simulink model "Manipulator_4DOF_dynamics_001"  (R2021b)
settings: Solver=VariableStepAuto  StartTime=0.0  StopTime=10.0  RelTol=1e-3
settings Model: Creator=rusla  LastModifiedBy=rusla

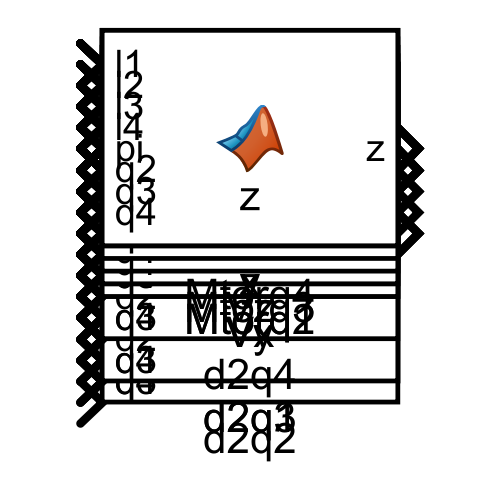
[thumbnail: Simulink's stored preview of the top-level diagram]
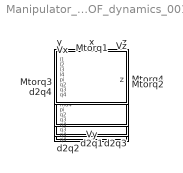
== system Manipulator_4DOF_dynamics_001 ==
  Mtorq1 : MATLAB Function  TreatAsAtomicUnit=on
  Mtorq2 : MATLAB Function  TreatAsAtomicUnit=on
  Mtorq3 : MATLAB Function  TreatAsAtomicUnit=on
  Mtorq4 : MATLAB Function  TreatAsAtomicUnit=on
  Vx : MATLAB Function  TreatAsAtomicUnit=on
  Vy : MATLAB Function  TreatAsAtomicUnit=on
  Vz : MATLAB Function  TreatAsAtomicUnit=on
  d2q1 : MATLAB Function  TreatAsAtomicUnit=on
  d2q2 : MATLAB Function  TreatAsAtomicUnit=on
  d2q3 : MATLAB Function  TreatAsAtomicUnit=on
  d2q4 : MATLAB Function  TreatAsAtomicUnit=on
  x : MATLAB Function  TreatAsAtomicUnit=on
  y : MATLAB Function  TreatAsAtomicUnit=on
  z : MATLAB Function  TreatAsAtomicUnit=on

== matlab function Manipulator_4DOF_dynamics_001/Vx ==
  data: dq1 input; Vx output; dq2 input; dq3 input; dq4 input; l2 input; l3 input; l4 input; pi input; q1 input; q2 input; q3 input; q4 input
function Vx = Vx(dq1,dq2,dq3,dq4,l2,l3,l4,pi,q1,q2,q3,q4)
%#codegen

%    This function was generated by the Symbolic Math Toolbox version 9.0.
%    11-May-2022 22:38:02

t2 = cos(q1);
t3 = cos(q2);
t4 = cos(q3);
t5 = cos(q4);
t6 = sin(q1);
t7 = sin(q2);
t8 = sin(q3);
t9 = sin(q4);
t14 = pi./2.0;
t10 = t2.*t3;
t11 = t2.*t7;
t12 = t3.*t6;
t13 = t6.*t7;
t15 = cos(t14);
t16 = t10.*t15;
t17 = t11.*t15;
t18 = t12.*t15;
t19 = t13.*t15;
t20 = -t17;
t21 = -t18;
t22 = t10+t19;
t23 = t13+t16;
t24 = t11+t21;
t25 = t12+t20;
t26 = t8.*t22;
t27 = t8.*t23;
t28 = t4.*t22;
t29 = t8.*t24;
t30 = t4.*t24;
t31 = t4.*t25;
t32 = -t30;
t33 = t27+t31;
t34 = t28+t29;
t35 = t26+t32;
t36 = t9.*t34;
t37 = l3.*t35;
t38 = t5.*t35;
t39 = t36+t38;
t40 = l4.*t39;
Vx = -dq3.*(t37+t40)-dq4.*t40+dq2.*(t37+t40-l2.*t24)-dq1.*(l4.*(t5.*t33+t9.*(t4.*t23-t8.*t25))+l2.*t25+l3.*t33);

== matlab function Manipulator_4DOF_dynamics_001/Vy ==
  data: dq1 input; Vy output; dq2 input; dq3 input; dq4 input; l2 input; l3 input; l4 input; pi input; q1 input; q2 input; q3 input; q4 input
function Vy = Vy(dq1,dq2,dq3,dq4,l2,l3,l4,pi,q1,q2,q3,q4)
%#codegen

%    This function was generated by the Symbolic Math Toolbox version 9.0.
%    11-May-2022 22:38:03

t2 = cos(q1);
t3 = cos(q2);
t4 = cos(q3);
t5 = cos(q4);
t6 = sin(q1);
t7 = sin(q2);
t8 = sin(q3);
t9 = sin(q4);
t14 = pi./2.0;
t10 = t2.*t3;
t11 = t2.*t7;
t12 = t3.*t6;
t13 = t6.*t7;
t15 = cos(t14);
t16 = t10.*t15;
t17 = t11.*t15;
t18 = t12.*t15;
t19 = t13.*t15;
t20 = -t17;
t21 = -t18;
t22 = t10+t19;
t23 = t13+t16;
t24 = t11+t21;
t25 = t12+t20;
t26 = t8.*t23;
t27 = t4.*t22;
t28 = t4.*t23;
t29 = t8.*t24;
t30 = t8.*t25;
t31 = t4.*t25;
t32 = -t28;
t33 = t26+t31;
t34 = t27+t29;
t35 = t30+t32;
t37 = -l3.*(t28-t30);
t38 = -t5.*(t28-t30);
t36 = t9.*t33;
t39 = t36+t38;
t40 = l4.*t39;
Vy = -dq3.*(t37+t40)-dq4.*t40-dq2.*(-t40+l2.*t23+l3.*(t28-t30))+dq1.*(l4.*(t5.*t34+t9.*(t4.*t24-t8.*t22))+l2.*t22+l3.*t34);

== matlab function Manipulator_4DOF_dynamics_001/Vz ==
  data: dq2 input; Vz output; dq3 input; dq4 input; l2 input; l3 input; l4 input; pi input; q2 input; q3 input; q4 input
function Vz = Vz(dq2,dq3,dq4,l2,l3,l4,pi,q2,q3,q4)
%#codegen

%    This function was generated by the Symbolic Math Toolbox version 9.0.
%    11-May-2022 22:38:04

t2 = -q2;
t3 = -q3;
t4 = q2+t3;
t6 = q3+q4+t2;
t5 = cos(t4);
t7 = cos(t6);
Vz = sin(pi./2.0).*(dq2.*l2.*cos(q2)+dq2.*l3.*t5-dq3.*l3.*t5+dq2.*l4.*t7-dq3.*l4.*t7-dq4.*l4.*t7);

== matlab function Manipulator_4DOF_dynamics_001/Mtorq1 ==
  data: Fx input; Mtorq1 output; Fy input; Mfi input; l2 input; l3 input; l4 input; pi input; q1 input; q2 input; q3 input; q4 input
function Mtorq1 = Mtorq1(Fx,Fy,Mfi,l2,l3,l4,pi,q1,q2,q3,q4)
%#codegen

%    This function was generated by the Symbolic Math Toolbox version 9.0.
%    11-May-2022 22:38:05

t2 = cos(q1);
t3 = cos(q2);
t4 = cos(q3);
t5 = cos(q4);
t6 = sin(q1);
t7 = sin(q2);
t8 = sin(q3);
t9 = sin(q4);
t14 = pi./2.0;
t10 = t2.*t3;
t11 = t2.*t7;
t12 = t3.*t6;
t13 = t6.*t7;
t15 = cos(t14);
t16 = t10.*t15;
t17 = t11.*t15;
t18 = t12.*t15;
t19 = t13.*t15;
t20 = -t17;
t21 = -t18;
t22 = t10+t19;
t23 = t13+t16;
t24 = t11+t21;
t25 = t12+t20;
t26 = t8.*t23;
t27 = t4.*t22;
t28 = t8.*t24;
t29 = t4.*t25;
t30 = t26+t29;
t31 = t27+t28;
Mtorq1 = Mfi-Fx.*(l4.*(t5.*t30+t9.*(t4.*t23-t8.*t25))+l2.*t25+l3.*t30)+Fy.*(l4.*(t5.*t31+t9.*(t4.*t24-t8.*t22))+l2.*t22+l3.*t31);

== matlab function Manipulator_4DOF_dynamics_001/Mtorq2 ==
  data: Fx input; Mtorq2 output; Fy input; Fz input; l2 input; l3 input; l4 input; pi input; q1 input; q2 input; q3 input; q4 input
function Mtorq2 = Mtorq2(Fx,Fy,Fz,l2,l3,l4,pi,q1,q2,q3,q4)
%#codegen

%    This function was generated by the Symbolic Math Toolbox version 9.0.
%    11-May-2022 22:38:06

t2 = cos(q1);
t3 = cos(q2);
t4 = cos(q3);
t5 = cos(q4);
t6 = sin(q1);
t7 = sin(q2);
t8 = sin(q3);
t9 = sin(q4);
t10 = -q3;
t15 = pi./2.0;
t11 = t2.*t3;
t12 = t2.*t7;
t13 = t3.*t6;
t14 = t6.*t7;
t16 = cos(t15);
t17 = sin(t15);
t18 = q2+t10;
t19 = t11.*t16;
t20 = t12.*t16;
t21 = t13.*t16;
t22 = t14.*t16;
t23 = -t20;
t24 = -t21;
t25 = t11+t22;
t26 = t14+t19;
t27 = t12+t24;
t28 = t13+t23;
t29 = t8.*t25;
t30 = t4.*t26;
t31 = t8.*t28;
t32 = t4.*t27;
t33 = -t30;
t34 = -t32;
t36 = t31+t33;
t35 = t29+t34;
Mtorq2 = -Fy.*(l2.*t26+l4.*(t5.*(t30-t31)-t9.*(t4.*t28+t8.*t26))+l3.*(t30-t31))+Fx.*(l4.*(t5.*t35+t9.*(t4.*t25+t8.*t27))-l2.*t27+l3.*t35)+Fz.*(l4.*(t5.*t17.*cos(t18)+t9.*t17.*sin(t18))+l3.*(t3.*t4.*t17+t7.*t8.*t17)+l2.*t3.*t17);

== matlab function Manipulator_4DOF_dynamics_001/Mtorq3 ==
  data: Fx input; Mtorq3 output; Fy input; Fz input; l3 input; l4 input; pi input; q1 input; q2 input; q3 input; q4 input
function Mtorq3 = Mtorq3(Fx,Fy,Fz,l3,l4,pi,q1,q2,q3,q4)
%#codegen

%    This function was generated by the Symbolic Math Toolbox version 9.0.
%    11-May-2022 22:38:07

t2 = cos(q1);
t3 = cos(q2);
t4 = cos(q3);
t5 = cos(q4);
t6 = sin(q1);
t7 = sin(q2);
t8 = sin(q3);
t9 = sin(q4);
t10 = -q3;
t15 = pi./2.0;
t11 = t2.*t3;
t12 = t2.*t7;
t13 = t3.*t6;
t14 = t6.*t7;
t16 = cos(t15);
t17 = sin(t15);
t18 = q2+t10;
t19 = t11.*t16;
t20 = t12.*t16;
t21 = t13.*t16;
t22 = t14.*t16;
t23 = -t20;
t24 = -t21;
t25 = t11+t22;
t26 = t14+t19;
t27 = t12+t24;
t28 = t13+t23;
t29 = t8.*t25;
t30 = t4.*t26;
t31 = t8.*t28;
t32 = t4.*t27;
t33 = -t30;
t34 = -t32;
t36 = t31+t33;
t35 = t29+t34;
Mtorq3 = -Fz.*(l4.*(t5.*t17.*cos(t18)+t9.*t17.*sin(t18))+l3.*(t3.*t4.*t17+t7.*t8.*t17))-Fx.*(l4.*(t5.*t35+t9.*(t4.*t25+t8.*t27))+l3.*t35)+Fy.*(l4.*(t5.*(t30-t31)-t9.*(t4.*t28+t8.*t26))+l3.*(t30-t31));

== matlab function Manipulator_4DOF_dynamics_001/Mtorq4 ==
  data: Fx input; Mtorq4 output; Fy input; Fz input; l4 input; pi input; q1 input; q2 input; q3 input; q4 input
function Mtorq4 = Mtorq4(Fx,Fy,Fz,l4,pi,q1,q2,q3,q4)
%#codegen

%    This function was generated by the Symbolic Math Toolbox version 9.0.
%    11-May-2022 22:38:08

t2 = cos(q1);
t3 = cos(q2);
t4 = cos(q3);
t5 = cos(q4);
t6 = sin(q1);
t7 = sin(q2);
t8 = sin(q3);
t9 = sin(q4);
t10 = -q3;
t15 = pi./2.0;
t11 = t2.*t3;
t12 = t2.*t7;
t13 = t3.*t6;
t14 = t6.*t7;
t16 = cos(t15);
t17 = sin(t15);
t18 = q2+t10;
t19 = t11.*t16;
t20 = t12.*t16;
t21 = t13.*t16;
t22 = t14.*t16;
t23 = -t20;
t24 = -t21;
t25 = t11+t22;
t26 = t14+t19;
t27 = t12+t24;
t28 = t13+t23;
Mtorq4 = -Fz.*l4.*(t5.*t17.*cos(t18)+t9.*t17.*sin(t18))+Fx.*l4.*(t5.*(t4.*t27-t8.*t25)-t9.*(t4.*t25+t8.*t27))+Fy.*l4.*(t5.*(t4.*t26-t8.*t28)-t9.*(t4.*t28+t8.*t26));

== matlab function Manipulator_4DOF_dynamics_001/x ==
  data: l2 input; x output; l3 input; l4 input; pi input; q1 input; q2 input; q3 input; q4 input
function x = x(l2,l3,l4,pi,q1,q2,q3,q4)
%#codegen

%    This function was generated by the Symbolic Math Toolbox version 9.0.
%    11-May-2022 22:38:09

t2 = cos(q1);
t3 = cos(q2);
t4 = cos(q3);
t5 = sin(q1);
t6 = sin(q2);
t7 = sin(q3);
t10 = pi./2.0;
t8 = t2.*t3;
t9 = t2.*t6;
t11 = cos(t10);
t12 = t3.*t5.*t11;
t13 = t5.*t6.*t11;
t14 = -t12;
t15 = t8+t13;
t16 = t9+t14;
t17 = t4.*t15;
t18 = t7.*t16;
t19 = t17+t18;
x = l4.*(sin(q4).*(t4.*t16-t7.*t15)+t19.*cos(q4))+l2.*t15+l3.*t19;

== matlab function Manipulator_4DOF_dynamics_001/d2q2 ==
  data: B input; d2q2 output; dq1 input; dq2 input; dq3 input; dq4 input; g input; l2 input; l3 input; l4 input; m2 input; m3 input; m4 input; mu2 input; pi input; q2 input; q3 input; q4 input
function d2q2 = d2q2(B,dq1,dq2,dq3,dq4,g,l2,l3,l4,m2,m3,m4,mu2,pi,q2,q3,q4)
%#codegen

%    This function was generated by the Symbolic Math Toolbox version 9.0.
%    11-May-2022 22:37:59

t2 = cos(q2);
t3 = sin(q3);
t4 = sin(q4);
t5 = B+q4;
t6 = q3+q4;
t7 = B.*2.0;
t8 = dq1.^2;
t9 = dq3.^2;
t10 = dq4.^2;
t11 = l2.^2;
t12 = l3.^2;
t13 = l4.^2;
t14 = q2.*2.0;
t15 = q3.*2.0;
t16 = q4.*2.0;
t21 = -pi;
t22 = -q2;
t24 = -q3;
t26 = -q4;
t28 = pi./2.0;
t17 = sin(t14);
t18 = q3+t5;
t19 = sin(t5);
t20 = sin(t6);
t23 = -t14;
t25 = -t15;
t27 = pi+t14;
t31 = cos(t28);
t32 = sin(t28);
t34 = q2+t24;
t38 = t14+t24;
t29 = sin(t18);
t30 = sin(t27);
t33 = pi+t23;
t35 = cos(t34);
t39 = t14+t25;
t41 = t24+t27;
t43 = t25+t27;
t44 = sin(t38);
t36 = q3+t33;
t37 = sin(t33);
t42 = t15+t33;
t45 = sin(t39);
t46 = sin(t41);
t48 = sin(t43);
t40 = sin(t36);
t47 = sin(t42);
et1 = mu2.*4.0-(m2.*t8.*t11.*t17)./3.0-m3.*t8.*t11.*t17-m4.*t8.*t11.*t17+(m2.*t8.*t11.*t30)./6.0+(m3.*t8.*t11.*t30)./2.0+(m4.*t8.*t11.*t30)./2.0-(m2.*t8.*t11.*t37)./6.0-(m3.*t8.*t11.*t37)./2.0-(m4.*t8.*t11.*t37)./2.0-(m3.*t8.*t12.*t45)./3.0-m4.*t8.*t12.*t45-(m3.*t8.*t12.*t47)./6.0+(m3.*t8.*t12.*t48)./6.0-(m4.*t8.*t12.*t47)./2.0+(m4.*t8.*t12.*t48)./2.0+(m4.*t8.*t13.*sin(t5.*2.0+t15+t23))./3.0+(m4.*t8.*t13.*sin(t6+t18+t21+t23))./2.0-(m4.*t8.*t13.*sin(t5.*2.0+t15+t21+t23))./6.0+m4.*t8.*t13.*sin(t6.*2.0+t23)+(m4.*t8.*t13.*sin(t6.*-2.0+t27))./2.0;
et2 = m4.*t8.*t13.*sin(t6.*2.0+t33).*(-1.0./2.0)-(m4.*t8.*t13.*sin(t5.*2.0+t42))./6.0-m4.*t8.*t13.*sin(t6+t18+t23)+(m4.*t8.*t13.*sin(t6+t18+t33))./2.0+l2.*l4.*m4.*t8.*sin(-t6+t27)+l3.*l4.*m4.*t8.*sin(-t6+t41)+l3.*l4.*m4.*t8.*sin(q3+t6+t23).*2.0-l3.*l4.*m4.*t8.*sin(t5+t15+t23)+(l2.*l4.*m4.*t8.*sin(t18+t21+t23))./2.0-g.*l2.*m2.*t2.*t32.*2.0-g.*l2.*m3.*t2.*t32.*4.0-g.*l2.*m4.*t2.*t32.*4.0-g.*l3.*m3.*t32.*t35.*2.0-g.*l3.*m4.*t32.*t35.*4.0-l2.*l3.*m3.*t3.*t9.*2.0-l2.*l3.*m4.*t3.*t9.*4.0-l3.*l4.*m4.*t4.*t10.*4.0-l2.*l4.*m4.*t9.*t20.*4.0-l2.*l4.*m4.*t10.*t20.*4.0+l3.*l4.*m4.*t10.*t19.*2.0;
et3 = l2.*l4.*m4.*t9.*t29.*2.0+l2.*l4.*m4.*t10.*t29.*2.0-(l2.*l3.*m3.*t8.*t40)./2.0-l2.*l3.*m4.*t8.*t40-l2.*l3.*m3.*t8.*t44-l2.*l3.*m4.*t8.*t44.*2.0+(l2.*l3.*m3.*t8.*t46)./2.0+l2.*l3.*m4.*t8.*t46+(l3.*l4.*m4.*t8.*sin(t5+t15+t21+t23))./2.0-g.*l4.*m4.*t32.*cos(t6+t22).*4.0+g.*l4.*m4.*t32.*cos(t18+t22).*2.0+l2.*l4.*m4.*t8.*sin(t6+t23).*2.0-l2.*l4.*m4.*t8.*sin(t6+t33)-l2.*l4.*m4.*t8.*sin(t18+t23)-l3.*l4.*m4.*t8.*sin(t6+t36)+(l3.*l4.*m4.*t8.*sin(t5+t42))./2.0+(l2.*l4.*m4.*t8.*sin(t18+t33))./2.0+dq2.*dq3.*l2.*l3.*m3.*t3.*4.0+dq2.*dq3.*l2.*l3.*m4.*t3.*8.0+dq2.*dq4.*l3.*l4.*m4.*t4.*8.0;
et4 = dq3.*dq4.*l3.*l4.*m4.*t4.*-8.0+dq2.*dq3.*l2.*l4.*m4.*t20.*8.0+dq2.*dq4.*l2.*l4.*m4.*t20.*8.0-dq2.*dq4.*l3.*l4.*m4.*t19.*4.0-dq3.*dq4.*l2.*l4.*m4.*t20.*8.0+dq3.*dq4.*l3.*l4.*m4.*t19.*4.0-dq2.*dq3.*l2.*l4.*m4.*t29.*4.0-dq2.*dq4.*l2.*l4.*m4.*t29.*4.0+dq3.*dq4.*l2.*l4.*m4.*t29.*4.0-dq1.*dq3.*l2.*l3.*m3.*t3.*t31.*4.0-dq1.*dq3.*l2.*l3.*m4.*t3.*t31.*8.0-dq1.*dq4.*l3.*l4.*m4.*t4.*t31.*8.0-dq1.*dq3.*l2.*l4.*m4.*t20.*t31.*8.0-dq1.*dq4.*l2.*l4.*m4.*t20.*t31.*8.0+dq1.*dq4.*l3.*l4.*m4.*t19.*t31.*4.0+dq1.*dq3.*l2.*l4.*m4.*t29.*t31.*4.0+dq1.*dq4.*l2.*l4.*m4.*t29.*t31.*4.0;
d2q2 = et1+et2+et3+et4;

== matlab function Manipulator_4DOF_dynamics_001/y ==
  data: l2 input; y output; l3 input; l4 input; pi input; q1 input; q2 input; q3 input; q4 input
function y = y(l2,l3,l4,pi,q1,q2,q3,q4)
%#codegen

%    This function was generated by the Symbolic Math Toolbox version 9.0.
%    11-May-2022 22:38:10

t2 = cos(q1);
t3 = cos(q2);
t4 = cos(q3);
t5 = sin(q1);
t6 = sin(q2);
t7 = sin(q3);
t10 = pi./2.0;
t8 = t3.*t5;
t9 = t5.*t6;
t11 = cos(t10);
t12 = t2.*t3.*t11;
t13 = t2.*t6.*t11;
t14 = -t13;
t15 = t9+t12;
t16 = t8+t14;
t17 = t7.*t15;
t18 = t4.*t16;
t19 = t17+t18;
y = l4.*(sin(q4).*(t4.*t15-t7.*t16)+t19.*cos(q4))+l2.*t16+l3.*t19;

== matlab function Manipulator_4DOF_dynamics_001/z ==
  data: l1 input; z output; l2 input; l3 input; l4 input; pi input; q2 input; q3 input; q4 input
function z = z(l1,l2,l3,l4,pi,q2,q3,q4)
%#codegen

%    This function was generated by the Symbolic Math Toolbox version 9.0.
%    11-May-2022 22:38:10

t2 = sin(q2);
t3 = -q3;
t4 = pi./2.0;
t5 = sin(t4);
t6 = q2+t3;
z = l1+l4.*(t5.*cos(q4).*sin(t6)-t5.*cos(t6).*sin(q4))+l3.*(t2.*t5.*cos(q3)-t5.*cos(q2).*sin(q3))+l2.*t2.*t5;

== matlab function Manipulator_4DOF_dynamics_001/d2q1 ==
  data: B input; d2q1 output; dq1 input; dq2 input; dq3 input; dq4 input; l2 input; l3 input; l4 input; m2 input; m3 input; m4 input; mu1 input; pi input; q2 input; q3 input; q4 input
function d2q1 = d2q1(B,dq1,dq2,dq3,dq4,l2,l3,l4,m2,m3,m4,mu1,pi,q2,q3,q4)
%#codegen

%    This function was generated by the Symbolic Math Toolbox version 9.0.
%    11-May-2022 22:37:55

t2 = sin(q3);
t3 = sin(q4);
t4 = B+q4;
t5 = pi+q3;
t6 = q3+q4;
t7 = B.*2.0;
t8 = dq3.^2;
t9 = l2.^2;
t10 = l3.^2;
t11 = l4.^2;
t12 = q2.*2.0;
t13 = q3.*2.0;
t14 = q4.*2.0;
t21 = -pi;
t23 = -q3;
t25 = -q4;
t29 = pi./2.0;
t15 = sin(t12);
t16 = q3+t4;
t17 = sin(t4);
t18 = q4+t5;
t19 = sin(t5);
t20 = sin(t6);
t22 = -t12;
t24 = -t13;
t26 = -t14;
t28 = pi+t12;
t30 = t4+t5;
t35 = pi+t23;
t36 = -t29;
t38 = t6+t21;
t42 = q3+t29;
t43 = q4+t29;
t44 = t12+t23;
t46 = t6+t29;
t55 = t4+t29;
t82 = t23+t29;
t83 = t25+t29;
t27 = sin(t18);
t31 = sin(t16);
t32 = sin(t28);
t33 = sin(t30);
t34 = pi+t22;
t37 = t5+t22;
t39 = t6+t22;
t41 = sin(t35);
t45 = t12+t24;
t47 = sin(t42);
t48 = sin(t43);
t49 = t16+t21;
t50 = t16+t22;
t51 = t18+t22;
t53 = sin(t38);
t56 = t6+t36;
t57 = t16+t29;
t58 = sin(t55);
t59 = t23+t28;
t61 = t24+t28;
t63 = sin(t44);
t65 = sin(t46);
t66 = t22+t30;
t69 = t4+t36;
t72 = t16+t36;
t75 = t4+t13+t22;
t87 = sin(t82);
t88 = sin(t83);
t96 = -t6+t28;
t40 = sin(t34);
t52 = sin(t37);
t54 = sin(t39);
t60 = q3+t37;
t62 = q3+t39;
t64 = sin(t45);
t67 = sin(t49);
t68 = sin(t50);
t70 = sin(t51);
t71 = sin(t66);
t73 = sin(t69);
t74 = sin(t56);
t76 = sin(t57);
t77 = t6+t37;
t78 = sin(t59);
t80 = sin(t61);
t84 = t16+t37;
t85 = sin(t75);
t89 = sin(t72);
t90 = t6+t39;
t91 = t16+t39;
t92 = t22+t49;
t93 = t18+t39;
t97 = -t6+t59;
t98 = -t6+t96;
t99 = t30+t39;
t103 = t4+t75;
t104 = t21+t75;
t105 = sin(t96);
t109 = t30+t50;
t113 = t38+t50;
t79 = sin(t60);
t81 = sin(t62);
t86 = sin(t77);
t94 = sin(t90);
t95 = sin(t84);
t100 = sin(t91);
t101 = sin(t92);
t102 = sin(t93);
t106 = sin(t97);
t107 = sin(t98);
t108 = sin(t99);
t110 = sin(t103);
t111 = sin(t104);
t112 = sin(t109);
t114 = sin(t113);
t115 = t21+t103;
t116 = sin(t115);
et1 = mu1.*4.0+dq4.^2.*l4.*m4.*cos(t29).*(l3.*t3.*2.0-l3.*t17+l2.*t20.*2.0-l2.*t31).*2.0+dq1.*dq2.*m2.*t9.*t15.*(2.0./3.0)+dq1.*dq2.*m3.*t9.*t15.*2.0+dq1.*dq2.*m4.*t9.*t15.*2.0-(dq1.*dq2.*m2.*t9.*t32)./3.0-dq1.*dq2.*m3.*t9.*t32-dq1.*dq2.*m4.*t9.*t32+(dq1.*dq2.*m2.*t9.*t40)./3.0+dq1.*dq2.*m3.*t9.*t40+dq1.*dq2.*m4.*t9.*t40+dq1.*dq2.*m3.*t10.*t64.*(2.0./3.0)+dq1.*dq2.*m4.*t10.*t64.*2.0-dq1.*dq3.*m3.*t10.*t64.*(2.0./3.0)-dq1.*dq3.*m4.*t10.*t64.*2.0+(dq1.*dq2.*m3.*t10.*t79)./3.0-(dq1.*dq2.*m3.*t10.*t80)./3.0+dq1.*dq2.*m4.*t10.*t79-(dq1.*dq3.*m3.*t10.*t79)./3.0-dq1.*dq2.*m4.*t10.*t80+(dq1.*dq3.*m3.*t10.*t80)./3.0-dq1.*dq3.*m4.*t10.*t79;
et2 = dq1.*dq3.*m4.*t10.*t80-dq1.*dq2.*m4.*t11.*t94.*2.0+dq1.*dq3.*m4.*t11.*t94.*2.0+dq1.*dq4.*m4.*t11.*t94.*2.0+dq1.*dq2.*m4.*t11.*t100.*2.0-dq1.*dq3.*m4.*t11.*t100.*2.0+dq1.*dq2.*m4.*t11.*t102-dq1.*dq4.*m4.*t11.*t100.*2.0-dq1.*dq3.*m4.*t11.*t102-dq1.*dq4.*m4.*t11.*t102-dq1.*dq2.*m4.*t11.*t107-dq1.*dq2.*m4.*t11.*t108+dq1.*dq3.*m4.*t11.*t107+dq1.*dq3.*m4.*t11.*t108+dq1.*dq4.*m4.*t11.*t107-dq1.*dq2.*m4.*t11.*t110.*(2.0./3.0)+dq1.*dq4.*m4.*t11.*t108+dq1.*dq3.*m4.*t11.*t110.*(2.0./3.0)+(dq1.*dq2.*m4.*t11.*t112)./3.0+dq1.*dq4.*m4.*t11.*t110.*(2.0./3.0)-(dq1.*dq3.*m4.*t11.*t112)./3.0-dq1.*dq2.*m4.*t11.*t114-(dq1.*dq4.*m4.*t11.*t112)./3.0+dq1.*dq3.*m4.*t11.*t114+(dq1.*dq2.*m4.*t11.*t116)./3.0+dq1.*dq4.*m4.*t11.*t114;
et3 = dq1.*dq3.*m4.*t11.*t116.*(-1.0./3.0)-(dq1.*dq4.*m4.*t11.*t116)./3.0+l2.*l3.*m3.*t8.*t47+l2.*l3.*m4.*t8.*t47.*2.0+l2.*l4.*m4.*t8.*t65.*2.0+l2.*l4.*m4.*t8.*t74.*2.0-l2.*l4.*m4.*t8.*t76-l2.*l3.*m3.*t8.*t87-l2.*l3.*m4.*t8.*t87.*2.0-l2.*l4.*m4.*t8.*t89+dq1.*dq4.*l3.*l4.*m4.*sin(pi+q4)-(dq1.*dq4.*l3.*l4.*m4.*sin(pi+t4))./2.0-dq1.*dq4.*l3.*l4.*m4.*sin(pi+t25)-(dq1.*dq4.*l3.*l4.*m4.*sin(t4+t21))./2.0+dq1.*dq3.*l2.*l3.*m3.*t2.*3.0+dq1.*dq3.*l2.*l3.*m4.*t2.*6.0+dq1.*dq4.*l3.*l4.*m4.*t3.*6.0+(dq1.*dq3.*l2.*l3.*m3.*t19)./2.0+dq1.*dq3.*l2.*l3.*m4.*t19-dq1.*dq4.*l3.*l4.*m4.*t17.*3.0+dq1.*dq3.*l2.*l4.*m4.*t20.*6.0+dq1.*dq4.*l2.*l4.*m4.*t20.*6.0;
et4 = dq1.*dq3.*l2.*l4.*m4.*t27+dq1.*dq4.*l2.*l4.*m4.*t27-dq1.*dq3.*l2.*l4.*m4.*t31.*3.0-dq1.*dq4.*l2.*l4.*m4.*t31.*3.0-(dq1.*dq3.*l2.*l4.*m4.*t33)./2.0-(dq1.*dq4.*l2.*l4.*m4.*t33)./2.0-(dq1.*dq3.*l2.*l3.*m3.*t41)./2.0-dq1.*dq3.*l2.*l3.*m4.*t41-dq2.*dq3.*l2.*l3.*m3.*t47.*2.0-dq2.*dq3.*l2.*l3.*m4.*t47.*4.0+dq1.*dq2.*l2.*l3.*m3.*t52+dq1.*dq2.*l2.*l3.*m4.*t52.*2.0-(dq1.*dq3.*l2.*l3.*m3.*t52)./2.0-dq1.*dq3.*l2.*l3.*m4.*t52-dq2.*dq4.*l3.*l4.*m4.*t48.*4.0+dq3.*dq4.*l3.*l4.*m4.*t48.*4.0-dq1.*dq2.*l2.*l4.*m4.*t54.*4.0+dq1.*dq3.*l2.*l4.*m4.*t53+dq1.*dq3.*l2.*l4.*m4.*t54.*2.0+dq1.*dq4.*l2.*l4.*m4.*t53+dq1.*dq4.*l2.*l4.*m4.*t54.*2.0+dq1.*dq2.*l2.*l3.*m3.*t63.*2.0+dq1.*dq2.*l2.*l3.*m4.*t63.*4.0;
et5 = -dq1.*dq3.*l2.*l3.*m3.*t63+dq2.*dq4.*l3.*l4.*m4.*t58.*2.0-dq1.*dq3.*l2.*l3.*m4.*t63.*2.0-dq3.*dq4.*l3.*l4.*m4.*t58.*2.0-dq2.*dq3.*l2.*l4.*m4.*t65.*4.0+dq1.*dq2.*l2.*l4.*m4.*t68.*2.0-(dq1.*dq3.*l2.*l4.*m4.*t67)./2.0-dq2.*dq4.*l2.*l4.*m4.*t65.*4.0-dq1.*dq3.*l2.*l4.*m4.*t68-(dq1.*dq4.*l2.*l4.*m4.*t67)./2.0+dq3.*dq4.*l2.*l4.*m4.*t65.*4.0+dq1.*dq2.*l2.*l4.*m4.*t70.*2.0-dq1.*dq4.*l2.*l4.*m4.*t68-dq1.*dq2.*l2.*l4.*m4.*t71-dq1.*dq3.*l2.*l4.*m4.*t70+(dq1.*dq3.*l2.*l4.*m4.*t71)./2.0-dq1.*dq4.*l2.*l4.*m4.*t70+(dq1.*dq4.*l2.*l4.*m4.*t71)./2.0-dq1.*dq2.*l2.*l3.*m3.*t78-dq2.*dq3.*l2.*l4.*m4.*t74.*4.0-dq1.*dq2.*l2.*l3.*m4.*t78.*2.0;
et6 = (dq1.*dq3.*l2.*l3.*m3.*t78)./2.0-dq2.*dq4.*l2.*l4.*m4.*t74.*4.0+dq2.*dq4.*l3.*l4.*m4.*t73.*2.0+dq1.*dq3.*l2.*l3.*m4.*t78+dq2.*dq3.*l2.*l4.*m4.*t76.*2.0+dq3.*dq4.*l2.*l4.*m4.*t74.*4.0-dq3.*dq4.*l3.*l4.*m4.*t73.*2.0+dq2.*dq4.*l2.*l4.*m4.*t76.*2.0-dq3.*dq4.*l2.*l4.*m4.*t76.*2.0-dq1.*dq2.*l3.*l4.*m4.*t81.*4.0+dq1.*dq3.*l3.*l4.*m4.*t81.*4.0+dq1.*dq4.*l3.*l4.*m4.*t81.*2.0+dq1.*dq2.*l3.*l4.*m4.*t85.*2.0+dq1.*dq2.*l3.*l4.*m4.*t86.*2.0-dq1.*dq3.*l3.*l4.*m4.*t85.*2.0+dq2.*dq3.*l2.*l3.*m3.*t87.*2.0-dq1.*dq3.*l3.*l4.*m4.*t86.*2.0-dq1.*dq4.*l3.*l4.*m4.*t85+dq2.*dq3.*l2.*l3.*m4.*t87.*4.0-dq1.*dq4.*l3.*l4.*m4.*t86+dq2.*dq3.*l2.*l4.*m4.*t89.*2.0+dq2.*dq4.*l2.*l4.*m4.*t89.*2.0+dq2.*dq4.*l3.*l4.*m4.*t88.*4.0;
et7 = dq3.*dq4.*l2.*l4.*m4.*t89.*-2.0-dq3.*dq4.*l3.*l4.*m4.*t88.*4.0-dq1.*dq2.*l3.*l4.*m4.*t95+dq1.*dq3.*l3.*l4.*m4.*t95+(dq1.*dq4.*l3.*l4.*m4.*t95)./2.0-dq1.*dq2.*l2.*l4.*m4.*t101+(dq1.*dq3.*l2.*l4.*m4.*t101)./2.0+(dq1.*dq4.*l2.*l4.*m4.*t101)./2.0-dq1.*dq2.*l2.*l4.*m4.*t105.*2.0+dq1.*dq3.*l2.*l4.*m4.*t105-dq1.*dq2.*l3.*l4.*m4.*t106.*2.0+dq1.*dq4.*l2.*l4.*m4.*t105+dq1.*dq3.*l3.*l4.*m4.*t106.*2.0+dq1.*dq4.*l3.*l4.*m4.*t106-dq1.*dq2.*l3.*l4.*m4.*t111+dq1.*dq3.*l3.*l4.*m4.*t111+(dq1.*dq4.*l3.*l4.*m4.*t111)./2.0;
d2q1 = et1+et2+et3+et4+et5+et6+et7;

== matlab function Manipulator_4DOF_dynamics_001/d2q3 ==
  data: B input; d2q3 output; dq1 input; dq2 input; dq3 input; dq4 input; g input; l2 input; l3 input; l4 input; m3 input; m4 input; mu3 input; pi input; q2 input; q3 input; q4 input
function d2q3 = d2q3(B,dq1,dq2,dq3,dq4,g,l2,l3,l4,m3,m4,mu3,pi,q2,q3,q4)
%#codegen

%    This function was generated by the Symbolic Math Toolbox version 9.0.
%    11-May-2022 22:38:00

t2 = sin(q3);
t3 = sin(q4);
t4 = B+q4;
t5 = pi+q3;
t6 = q3+q4;
t7 = B.*2.0;
t8 = dq1.^2;
t9 = dq2.^2;
t10 = dq4.^2;
t11 = l3.^2;
t12 = l4.^2;
t13 = q2.*2.0;
t14 = q3.*2.0;
t15 = q4.*2.0;
t20 = -pi;
t21 = -q2;
t23 = -q3;
t25 = -q4;
t26 = pi./2.0;
t16 = q3+t4;
t17 = sin(t4);
t18 = sin(t5);
t19 = sin(t6);
t22 = -t13;
t24 = -t14;
t28 = sin(t26);
t29 = pi+t23;
t30 = q2+t23;
t31 = -t26;
t35 = q3+t26;
t36 = t13+t23;
t48 = t23+t26;
t27 = sin(t16);
t32 = cos(t30);
t33 = t5+t22;
t34 = sin(t29);
t37 = t13+t24;
t38 = sin(t35);
t40 = t13+t29;
t43 = sin(t36);
t49 = sin(t48);
t39 = sin(t33);
t41 = q3+t33;
t42 = pi+t37;
t44 = sin(t37);
t45 = sin(t40);
t46 = sin(t41);
t47 = sin(t42);
et1 = mu3.*4.0+(m3.*t8.*t11.*t44)./3.0+m4.*t8.*t11.*t44+(m3.*t8.*t11.*t46)./6.0-(m3.*t8.*t11.*t47)./6.0+(m4.*t8.*t11.*t46)./2.0-(m4.*t8.*t11.*t47)./2.0-(m4.*t8.*t12.*sin(pi-t6.*2.0+t13))./2.0-(m4.*t8.*t12.*sin(t4.*2.0+t14+t22))./3.0-(m4.*t8.*t12.*sin(t6+t16+t20+t22))./2.0+(m4.*t8.*t12.*sin(t4.*2.0+t14+t20+t22))./6.0-m4.*t8.*t12.*sin(t6.*2.0+t22)+(m4.*t8.*t12.*sin(q4+t6+t33))./2.0-(m4.*t8.*t12.*sin(t4+t6+t33))./2.0+m4.*t8.*t12.*sin(t6+t16+t22)+(m4.*t8.*t12.*sin(t4+t16+t33))./6.0-l3.*l4.*m4.*t8.*sin(-t6+t40)-l3.*l4.*m4.*t8.*sin(q3+t6+t22).*2.0;
et2 = l3.*l4.*m4.*t8.*sin(t4+t14+t22)-(l2.*l4.*m4.*t8.*sin(t16+t20+t22))./4.0+g.*l3.*m3.*t28.*t32.*2.0+g.*l3.*m4.*t28.*t32.*4.0-l2.*l3.*m3.*t2.*t8.*(3.0./2.0)-l2.*l3.*m3.*t2.*t9.*2.0-l2.*l3.*m4.*t2.*t8.*3.0-l2.*l3.*m4.*t2.*t9.*4.0+l3.*l4.*m4.*t3.*t10.*4.0-(l2.*l3.*m3.*t8.*t18)./4.0-(l2.*l3.*m4.*t8.*t18)./2.0-l2.*l4.*m4.*t8.*t19.*3.0-l2.*l4.*m4.*t9.*t19.*4.0-l3.*l4.*m4.*t10.*t17.*2.0+l2.*l4.*m4.*t8.*t27.*(3.0./2.0)+l2.*l4.*m4.*t9.*t27.*2.0+(l2.*l3.*m3.*t8.*t34)./4.0+(l2.*l3.*m4.*t8.*t34)./2.0+(l2.*l3.*m3.*t8.*t39)./4.0+(l2.*l3.*m4.*t8.*t39)./2.0+(l2.*l3.*m3.*t8.*t43)./2.0+l2.*l3.*m4.*t8.*t43-(l2.*l3.*m3.*t8.*t45)./4.0;
et3 = l2.*l3.*m4.*t8.*t45.*(-1.0./2.0)-(l2.*l4.*m4.*t8.*sin(pi-t6+t13))./2.0-(l3.*l4.*m4.*t8.*sin(t4+t14+t20+t22))./2.0+g.*l4.*m4.*t28.*cos(t6+t21).*4.0-g.*l4.*m4.*t28.*cos(t16+t21).*2.0-(l2.*l4.*m4.*t8.*sin(q4+t5))./2.0+(l2.*l4.*m4.*t8.*sin(q4+t33))./2.0+(l2.*l4.*m4.*t8.*sin(t4+t5))./4.0-(l2.*l4.*m4.*t8.*sin(t6+t20))./2.0-l2.*l4.*m4.*t8.*sin(t6+t22)+(l2.*l4.*m4.*t8.*sin(t16+t20))./4.0-(l2.*l4.*m4.*t8.*sin(t4+t33))./4.0+(l2.*l4.*m4.*t8.*sin(t16+t22))./2.0+l3.*l4.*m4.*t8.*sin(t6+t33)-(l3.*l4.*m4.*t8.*sin(t16+t33))./2.0+dq1.*dq4.*l3.*l4.*m4.*sin(q4+t26).*4.0;
et4 = dq1.*dq2.*l2.*l4.*m4.*sin(t6+t26).*4.0-dq1.*dq4.*l3.*l4.*m4.*sin(t4+t26).*2.0+dq1.*dq2.*l2.*l4.*m4.*sin(t6+t31).*4.0-dq1.*dq4.*l3.*l4.*m4.*sin(t4+t31).*2.0-dq1.*dq2.*l2.*l4.*m4.*sin(t16+t26).*2.0-dq1.*dq2.*l2.*l4.*m4.*sin(t16+t31).*2.0-dq1.*dq4.*l3.*l4.*m4.*sin(t25+t26).*4.0-dq2.*dq4.*l3.*l4.*m4.*t3.*8.0+dq3.*dq4.*l3.*l4.*m4.*t3.*8.0+dq2.*dq4.*l3.*l4.*m4.*t17.*4.0-dq3.*dq4.*l3.*l4.*m4.*t17.*4.0+dq1.*dq2.*l2.*l3.*m3.*t38.*2.0+dq1.*dq2.*l2.*l3.*m4.*t38.*4.0-dq1.*dq2.*l2.*l3.*m3.*t49.*2.0-dq1.*dq2.*l2.*l3.*m4.*t49.*4.0;
d2q3 = et1+et2+et3+et4;

== matlab function Manipulator_4DOF_dynamics_001/d2q4 ==
  data: B input; d2q4 output; dq1 input; dq2 input; dq3 input; g input; l2 input; l3 input; l4 input; m4 input; mu4 input; pi input; q2 input; q3 input; q4 input
function d2q4 = d2q4(B,dq1,dq2,dq3,g,l2,l3,l4,m4,mu4,pi,q2,q3,q4)
%#codegen

%    This function was generated by the Symbolic Math Toolbox version 9.0.
%    11-May-2022 22:38:01

t2 = sin(q4);
t3 = B+q4;
t4 = q3+q4;
t5 = B.*2.0;
t6 = dq1.^2;
t7 = dq2.^2;
t8 = dq3.^2;
t9 = l4.^2;
t10 = q2.*2.0;
t11 = q3.*2.0;
t12 = q4.*2.0;
t16 = -pi;
t17 = -q2;
t19 = -q3;
t21 = -q4;
t22 = pi./2.0;
t13 = q3+t3;
t14 = sin(t3);
t15 = sin(t4);
t18 = -t10;
t20 = -t11;
t24 = -t22;
t25 = q4+t22;
t27 = t3+t22;
t31 = t21+t22;
t23 = sin(t13);
t26 = sin(t25);
t28 = sin(t27);
t29 = t3+t24;
t32 = sin(t31);
t30 = sin(t29);
et1 = mu4.*4.0+g.*l4.*m4.*sin(q2-t4+t22).*2.0-(m4.*t6.*t9.*sin(pi-t4.*2.0+t10))./2.0+(m4.*t6.*t9.*sin(pi+t4.*2.0+t18))./2.0-(m4.*t6.*t9.*sin(t3.*2.0+t11+t18))./3.0-(m4.*t6.*t9.*sin(pi+t4+t13+t18))./2.0-(m4.*t6.*t9.*sin(t4+t13+t16+t18))./2.0+(m4.*t6.*t9.*sin(pi+t3.*2.0+t11+t18))./6.0+(m4.*t6.*t9.*sin(t3.*2.0+t11+t16+t18))./6.0+g.*l4.*m4.*sin(t4+t17+t22).*2.0-g.*l4.*m4.*sin(t13+t17+t22)+g.*l4.*m4.*sin(t13+t17+t24)-m4.*t6.*t9.*sin(t4.*2.0+t18)+m4.*t6.*t9.*sin(t4+t13+t18)-(l3.*l4.*m4.*t6.*sin(pi-t4+t10+t19))./2.0;
et2 = (l2.*l4.*m4.*t6.*sin(pi+t4+t18))./2.0-(l2.*l4.*m4.*t6.*sin(pi+t13+t18))./4.0-l3.*l4.*m4.*t6.*sin(q3+t4+t18)+(l3.*l4.*m4.*t6.*sin(t3+t11+t18))./2.0-(l2.*l4.*m4.*t6.*sin(t13+t16+t18))./4.0-l3.*l4.*m4.*t2.*t6.*3.0-l3.*l4.*m4.*t2.*t7.*4.0-l3.*l4.*m4.*t2.*t8.*4.0-l2.*l4.*m4.*t6.*t15.*3.0+l3.*l4.*m4.*t6.*t14.*(3.0./2.0)-l2.*l4.*m4.*t7.*t15.*4.0+l3.*l4.*m4.*t7.*t14.*2.0+l3.*l4.*m4.*t8.*t14.*2.0+l2.*l4.*m4.*t6.*t23.*(3.0./2.0)+l2.*l4.*m4.*t7.*t23.*2.0-(l2.*l4.*m4.*t6.*sin(pi-t4+t10))./2.0+(l3.*l4.*m4.*t6.*sin(pi+q3+t4+t18))./2.0-(l3.*l4.*m4.*t6.*sin(pi+t3+t11+t18))./4.0;
et3 = l3.*l4.*m4.*t6.*sin(t3+t11+t16+t18).*(-1.0./4.0)-(l3.*l4.*m4.*t6.*sin(pi+q4))./2.0-(l2.*l4.*m4.*t6.*sin(pi+t4))./2.0+(l3.*l4.*m4.*t6.*sin(pi+t3))./4.0+(l2.*l4.*m4.*t6.*sin(pi+t13))./4.0+(l3.*l4.*m4.*t6.*sin(pi+t21))./2.0-(l2.*l4.*m4.*t6.*sin(t4+t16))./2.0+(l3.*l4.*m4.*t6.*sin(t3+t16))./4.0-l2.*l4.*m4.*t6.*sin(t4+t18)+(l2.*l4.*m4.*t6.*sin(t13+t16))./4.0+(l2.*l4.*m4.*t6.*sin(t13+t18))./2.0+dq1.*dq2.*l2.*l4.*m4.*sin(t4+t22).*4.0+dq1.*dq2.*l2.*l4.*m4.*sin(t4+t24).*4.0-dq1.*dq2.*l2.*l4.*m4.*sin(t13+t22).*2.0-dq1.*dq2.*l2.*l4.*m4.*sin(t13+t24).*2.0+dq2.*dq3.*l3.*l4.*m4.*t2.*8.0;
et4 = dq2.*dq3.*l3.*l4.*m4.*t14.*-4.0+dq1.*dq2.*l3.*l4.*m4.*t26.*4.0-dq1.*dq3.*l3.*l4.*m4.*t26.*4.0-dq1.*dq2.*l3.*l4.*m4.*t28.*2.0+dq1.*dq3.*l3.*l4.*m4.*t28.*2.0-dq1.*dq2.*l3.*l4.*m4.*t30.*2.0+dq1.*dq3.*l3.*l4.*m4.*t30.*2.0-dq1.*dq2.*l3.*l4.*m4.*t32.*4.0+dq1.*dq3.*l3.*l4.*m4.*t32.*4.0;
d2q4 = et1+et2+et3+et4;
